simulink model "uart_xy_wiggler"  (R2018a)
settings: Solver=FixedStepDiscrete  StartTime=0.0  StopTime=inf  RelTol=1e-3
PreLoadFcn:
  | waijung.modelPreload; % Required for working with Waijung Blockset. Do not remove.
undefined symbols (not defined in the file or in its folder): HSEOSC, Link, LQFP144, ST, STM32F446ZE
libraries: simulink x10, commsynccomp2 x7, stm32f4_io_lib x3, dspstat3 x2, stm32f4_device_config_lib x1, dspbuff3 x1
(part 9 of 9)

== system uart_xy_wiggler/set_UART_VCflag/Calibration Data Uart/Set UART vc Flag=5 ==
  UART Command : Inport
  Enable : EnablePort
  Volatile Data Storage Write : S-Function  FunctionName=waijung_vdata_write  Parameters=storagename,varname,sampletime,sampletimestr,blockid,storagetype,storagetypestr  SFunctionDeploymentMode=off  EnableBusSupport=off  mask(waijung_vdata_write){storagename=ab6, varname=CalibrationDataVolatileDataStorage4_ab6, sampletime=.01, sampletimestr=-1, blockid=set_UART_VCflagCalibrationDataUartSetUARTvcFlag5VolatileDataStorageWrite, storagetype=double, storagetypestr=double}
      mask prompts: storagename "Storage Name"; varname "Variable name"; sampletime "Sample time (sec)"; sampletimestr "Compiled sample time (sec) in string"; storagetype "Data type"; storagetypestr "Data type string"
      mask help: This block implements write data to a buffer.
      mask init:
      | waijung_vdata_write_callback('init');
      mask Help: web(fullfile(waijungdocroot,'Volatile_Data_Storage_Write.htm'))
      mask TypeOptions storagename: ab3 | ab1 | ab2 | ab4 | ab5 | ab6 | ab7 | ab8 | ab9 | ab10 | Ays | Ayc | Axs | A_Laser | LissaFreq | Axc | Laser | vcx | flag | CircleFlag | CircleFrequency | vcy | CircleR
      mask Callback storagename: waijung_vdata_write_callback('storagename');
      mask Callback varname: waijung_vdata_write_callback('varname');
      mask Callback sampletime: waijung_vdata_write_callback('sampletime');
      mask Callback sampletimestr: waijung_vdata_write_callback('sampletimestr');
      mask Callback blockid: waijung_vdata_write_callback('blockid');
      mask Callback storagetype: waijung_vdata_write_callback('storagetype');
      mask Display: text(0.95, 0.5, 'Buffer: ab6','ver','middle','hor','right');port_label('input',1,'D1(double)')
  wires:
  UART Command/1 -> Volatile Data Storage Write/1

== system uart_xy_wiggler/set_UART_VCflag/Calibration Data Uart/Set UART vc Flag=6 ==
  UART Command : Inport
  Enable : EnablePort
  Volatile Data Storage Write : S-Function  FunctionName=waijung_vdata_write  Parameters=storagename,varname,sampletime,sampletimestr,blockid,storagetype,storagetypestr  SFunctionDeploymentMode=off  EnableBusSupport=off  mask(waijung_vdata_write){storagename=ab7, varname=CalibrationDataVolatileDataStorage5_ab7, sampletime=.01, sampletimestr=-1, blockid=set_UART_VCflagCalibrationDataUartSetUARTvcFlag6VolatileDataStorageWrite, storagetype=double, storagetypestr=double}
      mask prompts: storagename "Storage Name"; varname "Variable name"; sampletime "Sample time (sec)"; sampletimestr "Compiled sample time (sec) in string"; storagetype "Data type"; storagetypestr "Data type string"
      mask help: This block implements write data to a buffer.
      mask init:
      | waijung_vdata_write_callback('init');
      mask Help: web(fullfile(waijungdocroot,'Volatile_Data_Storage_Write.htm'))
      mask TypeOptions storagename: ab3 | ab1 | ab2 | ab4 | ab5 | ab6 | ab7 | ab8 | ab9 | ab10 | Ays | Ayc | Axs | A_Laser | LissaFreq | Axc | Laser | vcx | flag | CircleFlag | CircleFrequency | vcy | CircleR
      mask Callback storagename: waijung_vdata_write_callback('storagename');
      mask Callback varname: waijung_vdata_write_callback('varname');
      mask Callback sampletime: waijung_vdata_write_callback('sampletime');
      mask Callback sampletimestr: waijung_vdata_write_callback('sampletimestr');
      mask Callback blockid: waijung_vdata_write_callback('blockid');
      mask Callback storagetype: waijung_vdata_write_callback('storagetype');
      mask Display: text(0.95, 0.5, 'Buffer: ab7','ver','middle','hor','right');port_label('input',1,'D1(double)')
  wires:
  UART Command/1 -> Volatile Data Storage Write/1

== system uart_xy_wiggler/set_UART_VCflag/Calibration Data Uart/Set UART vc Flag=7 ==
  UART Command : Inport
  Enable : EnablePort
  Volatile Data Storage Write : S-Function  FunctionName=waijung_vdata_write  Parameters=storagename,varname,sampletime,sampletimestr,blockid,storagetype,storagetypestr  SFunctionDeploymentMode=off  EnableBusSupport=off  mask(waijung_vdata_write){storagename=ab9, varname=CalibrationDataVolatileDataStorage7_ab9, sampletime=.01, sampletimestr=-1, blockid=set_UART_VCflagCalibrationDataUartSetUARTvcFlag7VolatileDataStorageWrite, storagetype=double, storagetypestr=double}
      mask prompts: storagename "Storage Name"; varname "Variable name"; sampletime "Sample time (sec)"; sampletimestr "Compiled sample time (sec) in string"; storagetype "Data type"; storagetypestr "Data type string"
      mask help: This block implements write data to a buffer.
      mask init:
      | waijung_vdata_write_callback('init');
      mask Help: web(fullfile(waijungdocroot,'Volatile_Data_Storage_Write.htm'))
      mask TypeOptions storagename: ab3 | ab1 | ab2 | ab4 | ab5 | ab6 | ab7 | ab8 | ab9 | ab10 | Ays | Ayc | Axs | A_Laser | LissaFreq | Axc | Laser | vcx | flag | CircleFlag | CircleFrequency | vcy | CircleR
      mask Callback storagename: waijung_vdata_write_callback('storagename');
      mask Callback varname: waijung_vdata_write_callback('varname');
      mask Callback sampletime: waijung_vdata_write_callback('sampletime');
      mask Callback sampletimestr: waijung_vdata_write_callback('sampletimestr');
      mask Callback blockid: waijung_vdata_write_callback('blockid');
      mask Callback storagetype: waijung_vdata_write_callback('storagetype');
      mask Display: text(0.95, 0.5, 'Buffer: ab9','ver','middle','hor','right');port_label('input',1,'D1(double)')
  wires:
  UART Command/1 -> Volatile Data Storage Write/1

== system uart_xy_wiggler/set_UART_VCflag/Calibration Data Uart/Set UART vc Flag=8 ==
  UART Command : Inport
  Enable : EnablePort
  Volatile Data Storage Write : S-Function  FunctionName=waijung_vdata_write  Parameters=storagename,varname,sampletime,sampletimestr,blockid,storagetype,storagetypestr  SFunctionDeploymentMode=off  EnableBusSupport=off  mask(waijung_vdata_write){storagename=ab10, varname=CalibrationDataVolatileDataStorage8_ab10, sampletime=.01, sampletimestr=-1, blockid=set_UART_VCflagCalibrationDataUartSetUARTvcFlag8VolatileDataStorageWrite, storagetype=double, storagetypestr=double}
      mask prompts: storagename "Storage Name"; varname "Variable name"; sampletime "Sample time (sec)"; sampletimestr "Compiled sample time (sec) in string"; storagetype "Data type"; storagetypestr "Data type string"
      mask help: This block implements write data to a buffer.
      mask init:
      | waijung_vdata_write_callback('init');
      mask Help: web(fullfile(waijungdocroot,'Volatile_Data_Storage_Write.htm'))
      mask TypeOptions storagename: ab3 | ab1 | ab2 | ab4 | ab5 | ab6 | ab7 | ab8 | ab9 | ab10 | Ays | Ayc | Axs | A_Laser | LissaFreq | Axc | Laser | vcx | flag | CircleFlag | CircleFrequency | vcy | CircleR
      mask Callback storagename: waijung_vdata_write_callback('storagename');
      mask Callback varname: waijung_vdata_write_callback('varname');
      mask Callback sampletime: waijung_vdata_write_callback('sampletime');
      mask Callback sampletimestr: waijung_vdata_write_callback('sampletimestr');
      mask Callback blockid: waijung_vdata_write_callback('blockid');
      mask Callback storagetype: waijung_vdata_write_callback('storagetype');
      mask Display: text(0.95, 0.5, 'Buffer: ab10','ver','middle','hor','right');port_label('input',1,'D1(double)')
  wires:
  UART Command/1 -> Volatile Data Storage Write/1

== system uart_xy_wiggler/set_UART_VCflag/Lissajous Data Uart/Set UART vc Flag=1 ==
  UART Command : Inport
  Enable : EnablePort
  Volatile Data Storage Write : S-Function  FunctionName=waijung_vdata_write  Parameters=storagename,varname,sampletime,sampletimestr,blockid,storagetype,storagetypestr  SFunctionDeploymentMode=off  EnableBusSupport=off  mask(waijung_vdata_write){storagename=A_Laser, varname=LissajousDataVolatileDataStorage7_A_Laser, sampletime=.01, sampletimestr=-1, blockid=set_UART_VCflagLissajousDataUartSetUARTvcFlag1VolatileDataStorageWrite, storagetype=double, storagetypestr=double}
      mask prompts: storagename "Storage Name"; varname "Variable name"; sampletime "Sample time (sec)"; sampletimestr "Compiled sample time (sec) in string"; storagetype "Data type"; storagetypestr "Data type string"
      mask help: This block implements write data to a buffer.
      mask init:
      | waijung_vdata_write_callback('init');
      mask Help: web(fullfile(waijungdocroot,'Volatile_Data_Storage_Write.htm'))
      mask TypeOptions storagename: ab3 | ab1 | ab2 | ab4 | ab5 | ab6 | ab7 | ab8 | ab9 | ab10 | Ays | Ayc | Axs | A_Laser | LissaFreq | Axc | Laser | vcx | flag | CircleFlag | CircleFrequency | vcy | CircleR
      mask Callback storagename: waijung_vdata_write_callback('storagename');
      mask Callback varname: waijung_vdata_write_callback('varname');
      mask Callback sampletime: waijung_vdata_write_callback('sampletime');
      mask Callback sampletimestr: waijung_vdata_write_callback('sampletimestr');
      mask Callback blockid: waijung_vdata_write_callback('blockid');
      mask Callback storagetype: waijung_vdata_write_callback('storagetype');
      mask Display: text(0.95, 0.5, 'Buffer: A_Laser','ver','middle','hor','right');port_label('input',1,'D1(double)')
  wires:
  UART Command/1 -> Volatile Data Storage Write/1

== system uart_xy_wiggler/set_UART_VCflag/Lissajous Data Uart/Set UART vc Flag=10 ==
  UART Command : Inport
  Enable : EnablePort
  Volatile Data Storage Write : S-Function  FunctionName=waijung_vdata_write  Parameters=storagename,varname,sampletime,sampletimestr,blockid,storagetype,storagetypestr  SFunctionDeploymentMode=off  EnableBusSupport=off  mask(waijung_vdata_write){storagename=Ayc, varname=LissajousDataVolatileDataStorage11_Ayc, sampletime=.01, sampletimestr=-1, blockid=set_UART_VCflagLissajousDataUartSetUARTvcFlag10VolatileDataStorageWrite, storagetype=double, storagetypestr=double}
      mask prompts: storagename "Storage Name"; varname "Variable name"; sampletime "Sample time (sec)"; sampletimestr "Compiled sample time (sec) in string"; storagetype "Data type"; storagetypestr "Data type string"
      mask help: This block implements write data to a buffer.
      mask init:
      | waijung_vdata_write_callback('init');
      mask Help: web(fullfile(waijungdocroot,'Volatile_Data_Storage_Write.htm'))
      mask TypeOptions storagename: ab3 | ab1 | ab2 | ab4 | ab5 | ab6 | ab7 | ab8 | ab9 | ab10 | Ays | Ayc | Axs | A_Laser | LissaFreq | Axc | Laser | vcx | flag | CircleFlag | CircleFrequency | vcy | CircleR
      mask Callback storagename: waijung_vdata_write_callback('storagename');
      mask Callback varname: waijung_vdata_write_callback('varname');
      mask Callback sampletime: waijung_vdata_write_callback('sampletime');
      mask Callback sampletimestr: waijung_vdata_write_callback('sampletimestr');
      mask Callback blockid: waijung_vdata_write_callback('blockid');
      mask Callback storagetype: waijung_vdata_write_callback('storagetype');
      mask Display: text(0.95, 0.5, 'Buffer: Ayc','ver','middle','hor','right');port_label('input',1,'D1(double)')
  wires:
  UART Command/1 -> Volatile Data Storage Write/1

== system uart_xy_wiggler/set_UART_VCflag/Lissajous Data Uart/Set UART vc Flag=11 ==
  UART Command : Inport
  Enable : EnablePort
  Volatile Data Storage Write : S-Function  FunctionName=waijung_vdata_write  Parameters=storagename,varname,sampletime,sampletimestr,blockid,storagetype,storagetypestr  SFunctionDeploymentMode=off  EnableBusSupport=off  mask(waijung_vdata_write){storagename=Axs, varname=LissajousDataVolatileDataStorage12_Axs, sampletime=.01, sampletimestr=-1, blockid=set_UART_VCflagLissajousDataUartSetUARTvcFlag11VolatileDataStorageWrite, storagetype=double, storagetypestr=double}
      mask prompts: storagename "Storage Name"; varname "Variable name"; sampletime "Sample time (sec)"; sampletimestr "Compiled sample time (sec) in string"; storagetype "Data type"; storagetypestr "Data type string"
      mask help: This block implements write data to a buffer.
      mask init:
      | waijung_vdata_write_callback('init');
      mask Help: web(fullfile(waijungdocroot,'Volatile_Data_Storage_Write.htm'))
      mask TypeOptions storagename: ab3 | ab1 | ab2 | ab4 | ab5 | ab6 | ab7 | ab8 | ab9 | ab10 | Ays | Ayc | Axs | A_Laser | LissaFreq | Axc | Laser | vcx | flag | CircleFlag | CircleFrequency | vcy | CircleR
      mask Callback storagename: waijung_vdata_write_callback('storagename');
      mask Callback varname: waijung_vdata_write_callback('varname');
      mask Callback sampletime: waijung_vdata_write_callback('sampletime');
      mask Callback sampletimestr: waijung_vdata_write_callback('sampletimestr');
      mask Callback blockid: waijung_vdata_write_callback('blockid');
      mask Callback storagetype: waijung_vdata_write_callback('storagetype');
      mask Display: text(0.95, 0.5, 'Buffer: Axs','ver','middle','hor','right');port_label('input',1,'D1(double)')
  wires:
  UART Command/1 -> Volatile Data Storage Write/1

== system uart_xy_wiggler/set_UART_VCflag/Lissajous Data Uart/Set UART vc Flag=7 ==
  UART Command : Inport
  Enable : EnablePort
  Volatile Data Storage Write : S-Function  FunctionName=waijung_vdata_write  Parameters=storagename,varname,sampletime,sampletimestr,blockid,storagetype,storagetypestr  SFunctionDeploymentMode=off  EnableBusSupport=off  mask(waijung_vdata_write){storagename=LissaFreq, varname=LissajousDataVolatileDataStorage8_LissaFreq, sampletime=.01, sampletimestr=-1, blockid=set_UART_VCflagLissajousDataUartSetUARTvcFlag7VolatileDataStorageWrite, storagetype=double, storagetypestr=double}
      mask prompts: storagename "Storage Name"; varname "Variable name"; sampletime "Sample time (sec)"; sampletimestr "Compiled sample time (sec) in string"; storagetype "Data type"; storagetypestr "Data type string"
      mask help: This block implements write data to a buffer.
      mask init:
      | waijung_vdata_write_callback('init');
      mask Help: web(fullfile(waijungdocroot,'Volatile_Data_Storage_Write.htm'))
      mask TypeOptions storagename: ab3 | ab1 | ab2 | ab4 | ab5 | ab6 | ab7 | ab8 | ab9 | ab10 | Ays | Ayc | Axs | A_Laser | LissaFreq | Axc | Laser | vcx | flag | CircleFlag | CircleFrequency | vcy | CircleR
      mask Callback storagename: waijung_vdata_write_callback('storagename');
      mask Callback varname: waijung_vdata_write_callback('varname');
      mask Callback sampletime: waijung_vdata_write_callback('sampletime');
      mask Callback sampletimestr: waijung_vdata_write_callback('sampletimestr');
      mask Callback blockid: waijung_vdata_write_callback('blockid');
      mask Callback storagetype: waijung_vdata_write_callback('storagetype');
      mask Display: text(0.95, 0.5, 'Buffer: LissaFreq','ver','middle','hor','right');port_label('input',1,'D1(double)')
  wires:
  UART Command/1 -> Volatile Data Storage Write/1

== system uart_xy_wiggler/set_UART_VCflag/Lissajous Data Uart/Set UART vc Flag=8 ==
  UART Command : Inport
  Enable : EnablePort
  Volatile Data Storage Write : S-Function  FunctionName=waijung_vdata_write  Parameters=storagename,varname,sampletime,sampletimestr,blockid,storagetype,storagetypestr  SFunctionDeploymentMode=off  EnableBusSupport=off  mask(waijung_vdata_write){storagename=Axc, varname=LissajousDataVolatileDataStorage9_Axc, sampletime=.01, sampletimestr=-1, blockid=set_UART_VCflagLissajousDataUartSetUARTvcFlag8VolatileDataStorageWrite, storagetype=double, storagetypestr=double}
      mask prompts: storagename "Storage Name"; varname "Variable name"; sampletime "Sample time (sec)"; sampletimestr "Compiled sample time (sec) in string"; storagetype "Data type"; storagetypestr "Data type string"
      mask help: This block implements write data to a buffer.
      mask init:
      | waijung_vdata_write_callback('init');
      mask Help: web(fullfile(waijungdocroot,'Volatile_Data_Storage_Write.htm'))
      mask TypeOptions storagename: ab3 | ab1 | ab2 | ab4 | ab5 | ab6 | ab7 | ab8 | ab9 | ab10 | Ays | Ayc | Axs | A_Laser | LissaFreq | Axc | Laser | vcx | flag | CircleFlag | CircleFrequency | vcy | CircleR
      mask Callback storagename: waijung_vdata_write_callback('storagename');
      mask Callback varname: waijung_vdata_write_callback('varname');
      mask Callback sampletime: waijung_vdata_write_callback('sampletime');
      mask Callback sampletimestr: waijung_vdata_write_callback('sampletimestr');
      mask Callback blockid: waijung_vdata_write_callback('blockid');
      mask Callback storagetype: waijung_vdata_write_callback('storagetype');
      mask Display: text(0.95, 0.5, 'Buffer: Axc','ver','middle','hor','right');port_label('input',1,'D1(double)')
  wires:
  UART Command/1 -> Volatile Data Storage Write/1

== system uart_xy_wiggler/set_UART_VCflag/Lissajous Data Uart/Set UART vc Flag=9 ==
  UART Command : Inport
  Enable : EnablePort
  Volatile Data Storage Write : S-Function  FunctionName=waijung_vdata_write  Parameters=storagename,varname,sampletime,sampletimestr,blockid,storagetype,storagetypestr  SFunctionDeploymentMode=off  EnableBusSupport=off  mask(waijung_vdata_write){storagename=Ays, varname=LissajousDataVolatileDataStorage10_Ays, sampletime=.01, sampletimestr=-1, blockid=set_UART_VCflagLissajousDataUartSetUARTvcFlag9VolatileDataStorageWrite, storagetype=double, storagetypestr=double}
      mask prompts: storagename "Storage Name"; varname "Variable name"; sampletime "Sample time (sec)"; sampletimestr "Compiled sample time (sec) in string"; storagetype "Data type"; storagetypestr "Data type string"
      mask help: This block implements write data to a buffer.
      mask init:
      | waijung_vdata_write_callback('init');
      mask Help: web(fullfile(waijungdocroot,'Volatile_Data_Storage_Write.htm'))
      mask TypeOptions storagename: ab3 | ab1 | ab2 | ab4 | ab5 | ab6 | ab7 | ab8 | ab9 | ab10 | Ays | Ayc | Axs | A_Laser | LissaFreq | Axc | Laser | vcx | flag | CircleFlag | CircleFrequency | vcy | CircleR
      mask Callback storagename: waijung_vdata_write_callback('storagename');
      mask Callback varname: waijung_vdata_write_callback('varname');
      mask Callback sampletime: waijung_vdata_write_callback('sampletime');
      mask Callback sampletimestr: waijung_vdata_write_callback('sampletimestr');
      mask Callback blockid: waijung_vdata_write_callback('blockid');
      mask Callback storagetype: waijung_vdata_write_callback('storagetype');
      mask Display: text(0.95, 0.5, 'Buffer: Ays','ver','middle','hor','right');port_label('input',1,'D1(double)')
  wires:
  UART Command/1 -> Volatile Data Storage Write/1
